simulink model "r2_deng_rev1_13_wide"  (R2012b)
settings: Solver=VariableStepDiscrete  StartTime=0.0  StopTime=2000  RelTol=1e-3
libraries: xbsIndex_r4 x7404, casper_library_sources x12, casper_library_misc x10, casper_library_communications x4, simulink x3, xps_library x2
(part 61 of 65)

== system r2_deng_rev1_13_wide/wng1/bus_mult/repb/bussify ==
  in1 : Inport
  in2 : Inport  Port=2
  in3 : Inport  Port=3
  in4 : Inport  Port=4
  in5 : Inport  Port=5
  in6 : Inport  Port=6
  in7 : Inport  Port=7
  in8 : Inport  Port=8
  concatenate : xbsIndex_r4/Concat  num_inputs=8  dbl_ovrd=off  block_type=concat
  reinterpret{1..8} (8 alike) : xbsIndex_r4/Reinterpret  force_arith_type=on  arith_type=Unsigned  force_bin_pt=on  bin_pt=0  block_type=reinterpret
      reinterpret1 settings: infoedit="Changes signal type without altering the binary representation.   You can changed the signal between signed and unsigned, and relocate the binary point.<br><br>Hardware notes: In hardware this block costs nothing.<br><br>Example:  Suppose the input is 6 bits wide, signed, with 2 fractional bits, and the output is forced to unsigned with 0 fractional bits.  Then an input of -2.0 (1110.00 in binary 2's complement) becomes an output of 56 (111000 in binary)."
  bus_out : Outport
  wires:
  concatenate/1 -> bus_out/1
  in1/1 -> reinterpret1/1
  reinterpret1/1 -> concatenate/1
  in2/1 -> reinterpret2/1
  reinterpret2/1 -> concatenate/2
  in3/1 -> reinterpret3/1
  reinterpret3/1 -> concatenate/3
  in4/1 -> reinterpret4/1
  reinterpret4/1 -> concatenate/4
  in5/1 -> reinterpret5/1
  reinterpret5/1 -> concatenate/5
  in6/1 -> reinterpret6/1
  reinterpret6/1 -> concatenate/6
  in7/1 -> reinterpret7/1
  reinterpret7/1 -> concatenate/7
  in8/1 -> reinterpret8/1
  reinterpret8/1 -> concatenate/8

== system r2_deng_rev1_13_wide/wng1/wgn1/tt800_uprng/tt800_engine ==
  note: Delay by (n - m - 3)
  note: Delay by (m)
  seed : Inport
  seed_en : Inport  Port=2
  Constant3 : xbsIndex_r4/Constant  const=0  gui_display_data_type=Fixed-point  arith_type=Unsigned  n_bits=32  bin_pt=0  preci_type=Single  exp_width=8  frac_width=24  explicit_period=off  period=1  equ=P=C  opselect=C  inp2=PCIN>>17  opr=+  inp1=P  carry=CIN  dbl_ovrd=off  block_type=constant
  Gateway Out{1..4} (4 alike) : xbsIndex_r4/Gateway Out  inherit_from_input=off  hdl_port=off  timing_constraint=None  locs_specified=off  LOCs={}  UseAsDAC=off  DACChannel='1'  block_type=gatewayout
      settings: infoedit="Gateway out block.  Converts Xilinx fixed point inputs into ouputs of type Simulink integer, double, or fixed point.<P><P>Hardware notes:  In hardware these blocks become top level output ports or are discarded, depending on how they are configured."  xl_area=[0 0 0 0 0 0 0]  block_version=10.1.3
  Logical : xbsIndex_r4/Logical  logical_function=XOR  inputs=3  en=off  latency=1  precision=Full  arith_type=Unsigned  n_bits=8  bin_pt=2  align_bp=off  dbl_ovrd=off  block_type=logical
      settings: xl_area=[32 32 0 32 0 0 0]
  Mux : xbsIndex_r4/Mux  inputs=2  en=off  latency=1  precision=Full  arith_type="Signed  (2's comp)"  n_bits=8  bin_pt=2  quantization=Truncate  overflow=Wrap  dbl_ovrd=off  block_type=mux
      settings: xl_area=[16 32 0 32 0 0 0]
  Mux1 : xbsIndex_r4/Mux  inputs=2  en=off  latency=1  precision=Full  arith_type="Signed  (2's comp)"  n_bits=8  bin_pt=2  quantization=Truncate  overflow=Wrap  dbl_ovrd=off  block_type=mux
      settings: xl_area=[16 32 0 32 0 0 0]
  Scope : Scope  NumInputPorts=4
      settings: YMin=-5~-5~-5~-5  YMax=5~5~5~5
  a : xbsIndex_r4/Constant  const=hex2dec('8EBFD028')  gui_display_data_type=Fixed-point  arith_type=Unsigned  n_bits=32  bin_pt=0  preci_type=Single  exp_width=8  frac_width=24  explicit_period=off  period=1  equ=P=C  opselect=C  inp2=PCIN>>17  opr=+  inp1=P  carry=CIN  dbl_ovrd=off  block_type=constant
  delay : xbsIndex_r4/Delay  rst=off  infoeditControl=Selection of Reset will increase slice count due to use of real FFs and instead of SRLs  en=off  latency=1  dbl_ovrd=off  reg_retiming=off  block_type=delay
      settings: xl_area=[16 32 0 0 0 0 0]
  lsb : xbsIndex_r4/Slice  nbits=1  boolean_output=off  mode=Lower Bit Location + Width  bit1=0  base1=MSB of Input  bit0=0  base0=LSB of Input  dbl_ovrd=off  block_type=slice
      settings: infoedit="Extracts a given range of bits from each input sample and presents it at the output.  The output type is ordinarily unsigned with binary point at zero, but can be Boolean when the slice is one bit wide.<P><P>Hardware notes: In hardware this block costs nothing."  block_version=10.1.3
  output : Subsystem
  rshift_1 : xbsIndex_r4/Shift  shift_dir=Right  shift_bits=1  en=off  latency=1  precision=User Defined  arith_type=Unsigned  n_bits=32  bin_pt=0  quantization=Truncate  overflow=Wrap  dbl_ovrd=off  block_type=shift
      settings: xl_area=[0 32 0 0 0 0 0]  block_version=10.1.3
  x_l : xbsIndex_r4/Delay  rst=off  infoeditControl=Selection of Reset will increase slice count due to use of real FFs and instead of SRLs  en=off  latency=7  dbl_ovrd=off  reg_retiming=off  block_type=delay
      settings: xl_area=[16 32 0 32 0 0 0]
  x_l_m : xbsIndex_r4/Delay  rst=off  infoeditControl=Selection of Reset will increase slice count due to use of real FFs and instead of SRLs  en=off  latency=25-7-3  dbl_ovrd=off  reg_retiming=off  block_type=delay
      settings: xl_area=[16 32 0 32 0 0 0]
  u : Outport
  wires:
  delay/1 -> Logical/1
  output/1(out) -> u/1
  Gateway Out3/1 -> Scope/4
  Gateway Out2/1 -> Scope/3
  Gateway Out4/1 -> Scope/2
  Gateway Out1/1 -> Scope/1
  seed/1 -> Mux1/3, Gateway Out4/1
  seed_en/1 -> Mux1/1, Gateway Out1/1
  Mux1/1 -> Gateway Out2/1, x_l_m/1
  Logical/1 -> Mux1/2, Gateway Out3/1
  Mux/1 -> Logical/3
  rshift_1/1 -> Logical/2
  a/1 -> Mux/3
  Constant3/1 -> Mux/2
  lsb/1 -> Mux/1
  x_l/1 -> output/1(in), rshift_1/1, lsb/1
  x_l_m/1 -> delay/1, x_l/1

== system r2_deng_rev1_13_wide/wng1/wgn1/tt800_uprng/tt800_seed_gen ==
  seed_in : Inport
  ld : Inport  Port=2
  rst : Inport  Port=3
  Expression : xbsIndex_r4/Expression  expression=(bootstrap | ld | ld_ext)  align_bp=on  en=off  latency=1  precision=Full  arith_type=Unsigned  n_bits=8  bin_pt=2  dbl_ovrd=off  block_type=expr
      settings: xl_area=[0, 0, 0, 0, 0, 0, 0]  block_version=10.1.3
  LFSR : xbsIndex_r4/LFSR  lfsr_type=Fibonacci  gate_type=XOR  n_bits=32  polynomial='C0000401'  rst_value='65498732'  rst=on  en=off  reloadable_seed=on  input_type=on  output_type=on  arith_type=Unsigned  bin_pt=0  dbl_ovrd=off  explicit_period=on  period=1  block_type=lfsr
      settings: xl_area=[17 32 0 33 0 0 0]  block_version=10.1.3
  bootstrap : Subsystem
  p24_extender : Subsystem
  pipeline1 : Subsystem  AncestorBlock=casper_library_delays/pipeline  mask(pipeline){latency=2}
      mask help:
      | An explicitly laid-out delay line to avoid mapping to SRL16s
      | for use in pipelining to help achieve timing closure.
      mask init:
      | pipeline_init(gcb,'latency',latency);
      settings: AttributesFormatString=Latency = %<latency>
      mask Display:
      | port_label('input', 1, 'd');
      | port_label('output', 1, 'q');
      | disp(['Z^-', num2str(latency)]);
  pipeline2 : Subsystem  AncestorBlock=casper_library_delays/pipeline  mask(pipeline){latency=2}
      mask help:
      | An explicitly laid-out delay line to avoid mapping to SRL16s
      | for use in pipelining to help achieve timing closure.
      mask init:
      | pipeline_init(gcb,'latency',latency);
      settings: AttributesFormatString=Latency = %<latency>
      mask Display:
      | port_label('input', 1, 'd');
      | port_label('output', 1, 'q');
      | disp(['Z^-', num2str(latency)]);
  r_edge_detect : Subsystem
  seed_out : Outport
  seed_en : Outport  Port=2
  wires:
  r_edge_detect/1(out) -> p24_extender/1(in)
  ld/1 -> LFSR/2, r_edge_detect/1(in), Expression/2
  Expression/1 -> seed_en/1
  seed_in/1 -> LFSR/1
  LFSR/1 -> seed_out/1
  bootstrap/1(out) -> Expression/1
  p24_extender/1(out) -> Expression/3
  rst/1 -> LFSR/3, pipeline2/1(d), pipeline1/1(d)
  pipeline2/1(q) -> p24_extender/2(rst)
  pipeline1/1(q) -> bootstrap/1(rst)

== system r2_deng_rev1_13_wide/wng1/wgn2/tt800_uprng/tt800_engine ==
  note: Delay by (n - m - 3)
  note: Delay by (m)
  seed : Inport
  seed_en : Inport  Port=2
  Constant3 : xbsIndex_r4/Constant  const=0  gui_display_data_type=Fixed-point  arith_type=Unsigned  n_bits=32  bin_pt=0  preci_type=Single  exp_width=8  frac_width=24  explicit_period=off  period=1  equ=P=C  opselect=C  inp2=PCIN>>17  opr=+  inp1=P  carry=CIN  dbl_ovrd=off  block_type=constant
  Gateway Out{1..4} (4 alike) : xbsIndex_r4/Gateway Out  inherit_from_input=off  hdl_port=off  timing_constraint=None  locs_specified=off  LOCs={}  UseAsDAC=off  DACChannel='1'  block_type=gatewayout
      settings: infoedit="Gateway out block.  Converts Xilinx fixed point inputs into ouputs of type Simulink integer, double, or fixed point.<P><P>Hardware notes:  In hardware these blocks become top level output ports or are discarded, depending on how they are configured."  xl_area=[0 0 0 0 0 0 0]  block_version=10.1.3
  Logical : xbsIndex_r4/Logical  logical_function=XOR  inputs=3  en=off  latency=1  precision=Full  arith_type=Unsigned  n_bits=8  bin_pt=2  align_bp=off  dbl_ovrd=off  block_type=logical
      settings: xl_area=[32 32 0 32 0 0 0]
  Mux : xbsIndex_r4/Mux  inputs=2  en=off  latency=1  precision=Full  arith_type="Signed  (2's comp)"  n_bits=8  bin_pt=2  quantization=Truncate  overflow=Wrap  dbl_ovrd=off  block_type=mux
      settings: xl_area=[16 32 0 32 0 0 0]
  Mux1 : xbsIndex_r4/Mux  inputs=2  en=off  latency=1  precision=Full  arith_type="Signed  (2's comp)"  n_bits=8  bin_pt=2  quantization=Truncate  overflow=Wrap  dbl_ovrd=off  block_type=mux
      settings: xl_area=[16 32 0 32 0 0 0]
  Scope : Scope  NumInputPorts=4
      settings: YMin=-5~-5~-5~-5  YMax=5~5~5~5
  a : xbsIndex_r4/Constant  const=hex2dec('8EBFD028')  gui_display_data_type=Fixed-point  arith_type=Unsigned  n_bits=32  bin_pt=0  preci_type=Single  exp_width=8  frac_width=24  explicit_period=off  period=1  equ=P=C  opselect=C  inp2=PCIN>>17  opr=+  inp1=P  carry=CIN  dbl_ovrd=off  block_type=constant
  delay : xbsIndex_r4/Delay  rst=off  infoeditControl=Selection of Reset will increase slice count due to use of real FFs and instead of SRLs  en=off  latency=1  dbl_ovrd=off  reg_retiming=off  block_type=delay
      settings: xl_area=[16 32 0 0 0 0 0]
  lsb : xbsIndex_r4/Slice  nbits=1  boolean_output=off  mode=Lower Bit Location + Width  bit1=0  base1=MSB of Input  bit0=0  base0=LSB of Input  dbl_ovrd=off  block_type=slice
      settings: infoedit="Extracts a given range of bits from each input sample and presents it at the output.  The output type is ordinarily unsigned with binary point at zero, but can be Boolean when the slice is one bit wide.<P><P>Hardware notes: In hardware this block costs nothing."  block_version=10.1.3
  output : Subsystem
  rshift_1 : xbsIndex_r4/Shift  shift_dir=Right  shift_bits=1  en=off  latency=1  precision=User Defined  arith_type=Unsigned  n_bits=32  bin_pt=0  quantization=Truncate  overflow=Wrap  dbl_ovrd=off  block_type=shift
      settings: xl_area=[0 32 0 0 0 0 0]  block_version=10.1.3
  x_l : xbsIndex_r4/Delay  rst=off  infoeditControl=Selection of Reset will increase slice count due to use of real FFs and instead of SRLs  en=off  latency=7  dbl_ovrd=off  reg_retiming=off  block_type=delay
      settings: xl_area=[16 32 0 32 0 0 0]
  x_l_m : xbsIndex_r4/Delay  rst=off  infoeditControl=Selection of Reset will increase slice count due to use of real FFs and instead of SRLs  en=off  latency=25-7-3  dbl_ovrd=off  reg_retiming=off  block_type=delay
      settings: xl_area=[16 32 0 32 0 0 0]
  u : Outport
  wires:
  delay/1 -> Logical/1
  output/1(out) -> u/1
  Gateway Out3/1 -> Scope/4
  Gateway Out2/1 -> Scope/3
  Gateway Out4/1 -> Scope/2
  Gateway Out1/1 -> Scope/1
  seed/1 -> Mux1/3, Gateway Out4/1
  seed_en/1 -> Mux1/1, Gateway Out1/1
  Mux1/1 -> Gateway Out2/1, x_l_m/1
  Logical/1 -> Mux1/2, Gateway Out3/1
  Mux/1 -> Logical/3
  rshift_1/1 -> Logical/2
  a/1 -> Mux/3
  Constant3/1 -> Mux/2
  lsb/1 -> Mux/1
  x_l/1 -> output/1(in), rshift_1/1, lsb/1
  x_l_m/1 -> delay/1, x_l/1

== system r2_deng_rev1_13_wide/wng1/wgn2/tt800_uprng/tt800_seed_gen ==
  seed_in : Inport
  ld : Inport  Port=2
  rst : Inport  Port=3
  Expression : xbsIndex_r4/Expression  expression=(bootstrap | ld | ld_ext)  align_bp=on  en=off  latency=1  precision=Full  arith_type=Unsigned  n_bits=8  bin_pt=2  dbl_ovrd=off  block_type=expr
      settings: xl_area=[0, 0, 0, 0, 0, 0, 0]  block_version=10.1.3
  LFSR : xbsIndex_r4/LFSR  lfsr_type=Fibonacci  gate_type=XOR  n_bits=32  polynomial='C0000401'  rst_value='32198754'  rst=on  en=off  reloadable_seed=on  input_type=on  output_type=on  arith_type=Unsigned  bin_pt=0  dbl_ovrd=off  explicit_period=on  period=1  block_type=lfsr
      settings: xl_area=[17 32 0 33 0 0 0]  block_version=10.1.3
  bootstrap : Subsystem
  p24_extender : Subsystem
  pipeline1 : Subsystem  AncestorBlock=casper_library_delays/pipeline  mask(pipeline){latency=2}
      mask help:
      | An explicitly laid-out delay line to avoid mapping to SRL16s
      | for use in pipelining to help achieve timing closure.
      mask init:
      | pipeline_init(gcb,'latency',latency);
      settings: AttributesFormatString=Latency = %<latency>
      mask Display:
      | port_label('input', 1, 'd');
      | port_label('output', 1, 'q');
      | disp(['Z^-', num2str(latency)]);
  pipeline2 : Subsystem  AncestorBlock=casper_library_delays/pipeline  mask(pipeline){latency=2}
      mask help:
      | An explicitly laid-out delay line to avoid mapping to SRL16s
      | for use in pipelining to help achieve timing closure.
      mask init:
      | pipeline_init(gcb,'latency',latency);
      settings: AttributesFormatString=Latency = %<latency>
      mask Display:
      | port_label('input', 1, 'd');
      | port_label('output', 1, 'q');
      | disp(['Z^-', num2str(latency)]);
  r_edge_detect : Subsystem
  seed_out : Outport
  seed_en : Outport  Port=2
  wires:
  r_edge_detect/1(out) -> p24_extender/1(in)
  ld/1 -> LFSR/2, r_edge_detect/1(in), Expression/2
  Expression/1 -> seed_en/1
  seed_in/1 -> LFSR/1
  LFSR/1 -> seed_out/1
  bootstrap/1(out) -> Expression/1
  p24_extender/1(out) -> Expression/3
  rst/1 -> pipeline1/1(d), pipeline2/1(d), LFSR/3
  pipeline1/1(q) -> p24_extender/2(rst)
  pipeline2/1(q) -> bootstrap/1(rst)

== system r2_deng_rev1_13_wide/wng1/wgn3/tt800_uprng/tt800_engine ==
  note: Delay by (n - m - 3)
  note: Delay by (m)
  seed : Inport
  seed_en : Inport  Port=2
  Constant3 : xbsIndex_r4/Constant  const=0  gui_display_data_type=Fixed-point  arith_type=Unsigned  n_bits=32  bin_pt=0  preci_type=Single  exp_width=8  frac_width=24  explicit_period=off  period=1  equ=P=C  opselect=C  inp2=PCIN>>17  opr=+  inp1=P  carry=CIN  dbl_ovrd=off  block_type=constant
  Gateway Out{1..4} (4 alike) : xbsIndex_r4/Gateway Out  inherit_from_input=off  hdl_port=off  timing_constraint=None  locs_specified=off  LOCs={}  UseAsDAC=off  DACChannel='1'  block_type=gatewayout
      settings: infoedit="Gateway out block.  Converts Xilinx fixed point inputs into ouputs of type Simulink integer, double, or fixed point.<P><P>Hardware notes:  In hardware these blocks become top level output ports or are discarded, depending on how they are configured."  xl_area=[0 0 0 0 0 0 0]  block_version=10.1.3
  Logical : xbsIndex_r4/Logical  logical_function=XOR  inputs=3  en=off  latency=1  precision=Full  arith_type=Unsigned  n_bits=8  bin_pt=2  align_bp=off  dbl_ovrd=off  block_type=logical
      settings: xl_area=[32 32 0 32 0 0 0]
  Mux : xbsIndex_r4/Mux  inputs=2  en=off  latency=1  precision=Full  arith_type="Signed  (2's comp)"  n_bits=8  bin_pt=2  quantization=Truncate  overflow=Wrap  dbl_ovrd=off  block_type=mux
      settings: xl_area=[16 32 0 32 0 0 0]
  Mux1 : xbsIndex_r4/Mux  inputs=2  en=off  latency=1  precision=Full  arith_type="Signed  (2's comp)"  n_bits=8  bin_pt=2  quantization=Truncate  overflow=Wrap  dbl_ovrd=off  block_type=mux
      settings: xl_area=[16 32 0 32 0 0 0]
  Scope : Scope  NumInputPorts=4
      settings: YMin=-5~-5~-5~-5  YMax=5~5~5~5
  a : xbsIndex_r4/Constant  const=hex2dec('8EBFD028')  gui_display_data_type=Fixed-point  arith_type=Unsigned  n_bits=32  bin_pt=0  preci_type=Single  exp_width=8  frac_width=24  explicit_period=off  period=1  equ=P=C  opselect=C  inp2=PCIN>>17  opr=+  inp1=P  carry=CIN  dbl_ovrd=off  block_type=constant
  delay : xbsIndex_r4/Delay  rst=off  infoeditControl=Selection of Reset will increase slice count due to use of real FFs and instead of SRLs  en=off  latency=1  dbl_ovrd=off  reg_retiming=off  block_type=delay
      settings: xl_area=[16 32 0 0 0 0 0]
  lsb : xbsIndex_r4/Slice  nbits=1  boolean_output=off  mode=Lower Bit Location + Width  bit1=0  base1=MSB of Input  bit0=0  base0=LSB of Input  dbl_ovrd=off  block_type=slice
      settings: infoedit="Extracts a given range of bits from each input sample and presents it at the output.  The output type is ordinarily unsigned with binary point at zero, but can be Boolean when the slice is one bit wide.<P><P>Hardware notes: In hardware this block costs nothing."  block_version=10.1.3
  output : Subsystem
  rshift_1 : xbsIndex_r4/Shift  shift_dir=Right  shift_bits=1  en=off  latency=1  precision=User Defined  arith_type=Unsigned  n_bits=32  bin_pt=0  quantization=Truncate  overflow=Wrap  dbl_ovrd=off  block_type=shift
      settings: xl_area=[0 32 0 0 0 0 0]  block_version=10.1.3
  x_l : xbsIndex_r4/Delay  rst=off  infoeditControl=Selection of Reset will increase slice count due to use of real FFs and instead of SRLs  en=off  latency=7  dbl_ovrd=off  reg_retiming=off  block_type=delay
      settings: xl_area=[16 32 0 32 0 0 0]
  x_l_m : xbsIndex_r4/Delay  rst=off  infoeditControl=Selection of Reset will increase slice count due to use of real FFs and instead of SRLs  en=off  latency=25-7-3  dbl_ovrd=off  reg_retiming=off  block_type=delay
      settings: xl_area=[16 32 0 32 0 0 0]
  u : Outport
  wires:
  delay/1 -> Logical/1
  output/1(out) -> u/1
  Gateway Out3/1 -> Scope/4
  Gateway Out2/1 -> Scope/3
  Gateway Out4/1 -> Scope/2
  Gateway Out1/1 -> Scope/1
  seed/1 -> Mux1/3, Gateway Out4/1
  seed_en/1 -> Mux1/1, Gateway Out1/1
  Mux1/1 -> Gateway Out2/1, x_l_m/1
  Logical/1 -> Mux1/2, Gateway Out3/1
  Mux/1 -> Logical/3
  rshift_1/1 -> Logical/2
  a/1 -> Mux/3
  Constant3/1 -> Mux/2
  lsb/1 -> Mux/1
  x_l/1 -> output/1(in), rshift_1/1, lsb/1
  x_l_m/1 -> delay/1, x_l/1

== system r2_deng_rev1_13_wide/wng1/wgn3/tt800_uprng/tt800_seed_gen ==
  seed_in : Inport
  ld : Inport  Port=2
  rst : Inport  Port=3
  Expression : xbsIndex_r4/Expression  expression=(bootstrap | ld | ld_ext)  align_bp=on  en=off  latency=1  precision=Full  arith_type=Unsigned  n_bits=8  bin_pt=2  dbl_ovrd=off  block_type=expr
      settings: xl_area=[0, 0, 0, 0, 0, 0, 0]  block_version=10.1.3
  LFSR : xbsIndex_r4/LFSR  lfsr_type=Fibonacci  gate_type=XOR  n_bits=32  polynomial='C0000401'  rst_value='45612378'  rst=on  en=off  reloadable_seed=on  input_type=on  output_type=on  arith_type=Unsigned  bin_pt=0  dbl_ovrd=off  explicit_period=on  period=1  block_type=lfsr
      settings: xl_area=[17 32 0 33 0 0 0]  block_version=10.1.3
  bootstrap : Subsystem
  p24_extender : Subsystem
  pipeline1 : Subsystem  AncestorBlock=casper_library_delays/pipeline  mask(pipeline){latency=2}
      mask help:
      | An explicitly laid-out delay line to avoid mapping to SRL16s
      | for use in pipelining to help achieve timing closure.
      mask init:
      | pipeline_init(gcb,'latency',latency);
      settings: AttributesFormatString=Latency = %<latency>
      mask Display:
      | port_label('input', 1, 'd');
      | port_label('output', 1, 'q');
      | disp(['Z^-', num2str(latency)]);
  pipeline2 : Subsystem  AncestorBlock=casper_library_delays/pipeline  mask(pipeline){latency=2}
      mask help:
      | An explicitly laid-out delay line to avoid mapping to SRL16s
      | for use in pipelining to help achieve timing closure.
      mask init:
      | pipeline_init(gcb,'latency',latency);
      settings: AttributesFormatString=Latency = %<latency>
      mask Display:
      | port_label('input', 1, 'd');
      | port_label('output', 1, 'q');
      | disp(['Z^-', num2str(latency)]);
  r_edge_detect : Subsystem
  seed_out : Outport
  seed_en : Outport  Port=2
  wires:
  r_edge_detect/1(out) -> p24_extender/1(in)
  ld/1 -> LFSR/2, r_edge_detect/1(in), Expression/2
  Expression/1 -> seed_en/1
  seed_in/1 -> LFSR/1
  LFSR/1 -> seed_out/1
  bootstrap/1(out) -> Expression/1
  p24_extender/1(out) -> Expression/3
  rst/1 -> pipeline1/1(d), pipeline2/1(d), LFSR/3
  pipeline1/1(q) -> p24_extender/2(rst)
  pipeline2/1(q) -> bootstrap/1(rst)

== system r2_deng_rev1_13_wide/wng1/wgn4/tt800_uprng/tt800_engine ==
  note: Delay by (n - m - 3)
  note: Delay by (m)
  seed : Inport
  seed_en : Inport  Port=2
  Constant3 : xbsIndex_r4/Constant  const=0  gui_display_data_type=Fixed-point  arith_type=Unsigned  n_bits=32  bin_pt=0  preci_type=Single  exp_width=8  frac_width=24  explicit_period=off  period=1  equ=P=C  opselect=C  inp2=PCIN>>17  opr=+  inp1=P  carry=CIN  dbl_ovrd=off  block_type=constant
  Gateway Out{1..4} (4 alike) : xbsIndex_r4/Gateway Out  inherit_from_input=off  hdl_port=off  timing_constraint=None  locs_specified=off  LOCs={}  UseAsDAC=off  DACChannel='1'  block_type=gatewayout
      settings: infoedit="Gateway out block.  Converts Xilinx fixed point inputs into ouputs of type Simulink integer, double, or fixed point.<P><P>Hardware notes:  In hardware these blocks become top level output ports or are discarded, depending on how they are configured."  xl_area=[0 0 0 0 0 0 0]  block_version=10.1.3
  Logical : xbsIndex_r4/Logical  logical_function=XOR  inputs=3  en=off  latency=1  precision=Full  arith_type=Unsigned  n_bits=8  bin_pt=2  align_bp=off  dbl_ovrd=off  block_type=logical
      settings: xl_area=[32 32 0 32 0 0 0]
  Mux : xbsIndex_r4/Mux  inputs=2  en=off  latency=1  precision=Full  arith_type="Signed  (2's comp)"  n_bits=8  bin_pt=2  quantization=Truncate  overflow=Wrap  dbl_ovrd=off  block_type=mux
      settings: xl_area=[16 32 0 32 0 0 0]
  Mux1 : xbsIndex_r4/Mux  inputs=2  en=off  latency=1  precision=Full  arith_type="Signed  (2's comp)"  n_bits=8  bin_pt=2  quantization=Truncate  overflow=Wrap  dbl_ovrd=off  block_type=mux
      settings: xl_area=[16 32 0 32 0 0 0]
  Scope : Scope  NumInputPorts=4
      settings: YMin=-5~-5~-5~-5  YMax=5~5~5~5
  a : xbsIndex_r4/Constant  const=hex2dec('8EBFD028')  gui_display_data_type=Fixed-point  arith_type=Unsigned  n_bits=32  bin_pt=0  preci_type=Single  exp_width=8  frac_width=24  explicit_period=off  period=1  equ=P=C  opselect=C  inp2=PCIN>>17  opr=+  inp1=P  carry=CIN  dbl_ovrd=off  block_type=constant
  delay : xbsIndex_r4/Delay  rst=off  infoeditControl=Selection of Reset will increase slice count due to use of real FFs and instead of SRLs  en=off  latency=1  dbl_ovrd=off  reg_retiming=off  block_type=delay
      settings: xl_area=[16 32 0 0 0 0 0]
  lsb : xbsIndex_r4/Slice  nbits=1  boolean_output=off  mode=Lower Bit Location + Width  bit1=0  base1=MSB of Input  bit0=0  base0=LSB of Input  dbl_ovrd=off  block_type=slice
      settings: infoedit="Extracts a given range of bits from each input sample and presents it at the output.  The output type is ordinarily unsigned with binary point at zero, but can be Boolean when the slice is one bit wide.<P><P>Hardware notes: In hardware this block costs nothing."  block_version=10.1.3
  output : Subsystem
  rshift_1 : xbsIndex_r4/Shift  shift_dir=Right  shift_bits=1  en=off  latency=1  precision=User Defined  arith_type=Unsigned  n_bits=32  bin_pt=0  quantization=Truncate  overflow=Wrap  dbl_ovrd=off  block_type=shift
      settings: xl_area=[0 32 0 0 0 0 0]  block_version=10.1.3
  x_l : xbsIndex_r4/Delay  rst=off  infoeditControl=Selection of Reset will increase slice count due to use of real FFs and instead of SRLs  en=off  latency=7  dbl_ovrd=off  reg_retiming=off  block_type=delay
      settings: xl_area=[16 32 0 32 0 0 0]
  x_l_m : xbsIndex_r4/Delay  rst=off  infoeditControl=Selection of Reset will increase slice count due to use of real FFs and instead of SRLs  en=off  latency=25-7-3  dbl_ovrd=off  reg_retiming=off  block_type=delay
      settings: xl_area=[16 32 0 32 0 0 0]
  u : Outport
  wires:
  delay/1 -> Logical/1
  output/1(out) -> u/1
  Gateway Out3/1 -> Scope/4
  Gateway Out2/1 -> Scope/3
  Gateway Out4/1 -> Scope/2
  Gateway Out1/1 -> Scope/1
  seed/1 -> Mux1/3, Gateway Out4/1
  seed_en/1 -> Mux1/1, Gateway Out1/1
  Mux1/1 -> Gateway Out2/1, x_l_m/1
  Logical/1 -> Mux1/2, Gateway Out3/1
  Mux/1 -> Logical/3
  rshift_1/1 -> Logical/2
  a/1 -> Mux/3
  Constant3/1 -> Mux/2
  lsb/1 -> Mux/1
  x_l/1 -> output/1(in), rshift_1/1, lsb/1
  x_l_m/1 -> delay/1, x_l/1

== system r2_deng_rev1_13_wide/wng1/wgn4/tt800_uprng/tt800_seed_gen ==
  seed_in : Inport
  ld : Inport  Port=2
  rst : Inport  Port=3
  Expression : xbsIndex_r4/Expression  expression=(bootstrap | ld | ld_ext)  align_bp=on  en=off  latency=1  precision=Full  arith_type=Unsigned  n_bits=8  bin_pt=2  dbl_ovrd=off  block_type=expr
      settings: xl_area=[0, 0, 0, 0, 0, 0, 0]  block_version=10.1.3
  LFSR : xbsIndex_r4/LFSR  lfsr_type=Fibonacci  gate_type=XOR  n_bits=32  polynomial='C0000401'  rst_value='74563218'  rst=on  en=off  reloadable_seed=on  input_type=on  output_type=on  arith_type=Unsigned  bin_pt=0  dbl_ovrd=off  explicit_period=on  period=1  block_type=lfsr
      settings: xl_area=[17 32 0 33 0 0 0]  block_version=10.1.3
  bootstrap : Subsystem
  p24_extender : Subsystem
  pipeline1 : Subsystem  AncestorBlock=casper_library_delays/pipeline  mask(pipeline){latency=2}
      mask help:
      | An explicitly laid-out delay line to avoid mapping to SRL16s
      | for use in pipelining to help achieve timing closure.
      mask init:
      | pipeline_init(gcb,'latency',latency);
      settings: AttributesFormatString=Latency = %<latency>
      mask Display:
      | port_label('input', 1, 'd');
      | port_label('output', 1, 'q');
      | disp(['Z^-', num2str(latency)]);
  pipeline2 : Subsystem  AncestorBlock=casper_library_delays/pipeline  mask(pipeline){latency=2}
      mask help:
      | An explicitly laid-out delay line to avoid mapping to SRL16s
      | for use in pipelining to help achieve timing closure.
      mask init:
      | pipeline_init(gcb,'latency',latency);
      settings: AttributesFormatString=Latency = %<latency>
      mask Display:
      | port_label('input', 1, 'd');
      | port_label('output', 1, 'q');
      | disp(['Z^-', num2str(latency)]);
  r_edge_detect : Subsystem
  seed_out : Outport
  seed_en : Outport  Port=2
  wires:
  r_edge_detect/1(out) -> p24_extender/1(in)
  ld/1 -> LFSR/2, r_edge_detect/1(in), Expression/2
  Expression/1 -> seed_en/1
  seed_in/1 -> LFSR/1
  LFSR/1 -> seed_out/1
  bootstrap/1(out) -> Expression/1
  p24_extender/1(out) -> Expression/3
  rst/1 -> LFSR/3, pipeline1/1(d), pipeline2/1(d)
  pipeline1/1(q) -> p24_extender/2(rst)
  pipeline2/1(q) -> bootstrap/1(rst)

== system r2_deng_rev1_13_wide/wng_corr/bus_mult/repa/bussify ==
  in1 : Inport
  reinterpret1 : xbsIndex_r4/Reinterpret  force_arith_type=on  arith_type=Unsigned  force_bin_pt=on  bin_pt=0  block_type=reinterpret
      settings: infoedit="Changes signal type without altering the binary representation.   You can changed the signal between signed and unsigned, and relocate the binary point.<br><br>Hardware notes: In hardware this block costs nothing.<br><br>Example:  Suppose the input is 6 bits wide, signed, with 2 fractional bits, and the output is forced to unsigned with 0 fractional bits.  Then an input of -2.0 (1110.00 in binary 2's complement) becomes an output of 56 (111000 in binary)."
  bus_out : Outport
  wires:
  in1/1 -> reinterpret1/1
  reinterpret1/1 -> bus_out/1

== system r2_deng_rev1_13_wide/wng_corr/bus_mult/repb/bussify ==
  in1 : Inport
  in2 : Inport  Port=2
  in3 : Inport  Port=3
  in4 : Inport  Port=4
  in5 : Inport  Port=5
  in6 : Inport  Port=6
  in7 : Inport  Port=7
  in8 : Inport  Port=8
  concatenate : xbsIndex_r4/Concat  num_inputs=8  dbl_ovrd=off  block_type=concat
  reinterpret{1..8} (8 alike) : xbsIndex_r4/Reinterpret  force_arith_type=on  arith_type=Unsigned  force_bin_pt=on  bin_pt=0  block_type=reinterpret
      reinterpret1 settings: infoedit="Changes signal type without altering the binary representation.   You can changed the signal between signed and unsigned, and relocate the binary point.<br><br>Hardware notes: In hardware this block costs nothing.<br><br>Example:  Suppose the input is 6 bits wide, signed, with 2 fractional bits, and the output is forced to unsigned with 0 fractional bits.  Then an input of -2.0 (1110.00 in binary 2's complement) becomes an output of 56 (111000 in binary)."
  bus_out : Outport
  wires:
  concatenate/1 -> bus_out/1
  in1/1 -> reinterpret1/1
  reinterpret1/1 -> concatenate/1
  in2/1 -> reinterpret2/1
  reinterpret2/1 -> concatenate/2
  in3/1 -> reinterpret3/1
  reinterpret3/1 -> concatenate/3
  in4/1 -> reinterpret4/1
  reinterpret4/1 -> concatenate/4
  in5/1 -> reinterpret5/1
  reinterpret5/1 -> concatenate/5
  in6/1 -> reinterpret6/1
  reinterpret6/1 -> concatenate/6
  in7/1 -> reinterpret7/1
  reinterpret7/1 -> concatenate/7
  in8/1 -> reinterpret8/1
  reinterpret8/1 -> concatenate/8

== system r2_deng_rev1_13_wide/wng_corr/wgn1/tt800_uprng/tt800_engine ==
  note: Delay by (n - m - 3)
  note: Delay by (m)
  seed : Inport
  seed_en : Inport  Port=2
  Constant3 : xbsIndex_r4/Constant  const=0  gui_display_data_type=Fixed-point  arith_type=Unsigned  n_bits=32  bin_pt=0  preci_type=Single  exp_width=8  frac_width=24  explicit_period=off  period=1  equ=P=C  opselect=C  inp2=PCIN>>17  opr=+  inp1=P  carry=CIN  dbl_ovrd=off  block_type=constant
  Gateway Out{1..4} (4 alike) : xbsIndex_r4/Gateway Out  inherit_from_input=off  hdl_port=off  timing_constraint=None  locs_specified=off  LOCs={}  UseAsDAC=off  DACChannel='1'  block_type=gatewayout
      settings: infoedit="Gateway out block.  Converts Xilinx fixed point inputs into ouputs of type Simulink integer, double, or fixed point.<P><P>Hardware notes:  In hardware these blocks become top level output ports or are discarded, depending on how they are configured."  xl_area=[0 0 0 0 0 0 0]  block_version=10.1.3
  Logical : xbsIndex_r4/Logical  logical_function=XOR  inputs=3  en=off  latency=1  precision=Full  arith_type=Unsigned  n_bits=8  bin_pt=2  align_bp=off  dbl_ovrd=off  block_type=logical
      settings: xl_area=[32 32 0 32 0 0 0]
  Mux : xbsIndex_r4/Mux  inputs=2  en=off  latency=1  precision=Full  arith_type="Signed  (2's comp)"  n_bits=8  bin_pt=2  quantization=Truncate  overflow=Wrap  dbl_ovrd=off  block_type=mux
      settings: xl_area=[16 32 0 32 0 0 0]
  Mux1 : xbsIndex_r4/Mux  inputs=2  en=off  latency=1  precision=Full  arith_type="Signed  (2's comp)"  n_bits=8  bin_pt=2  quantization=Truncate  overflow=Wrap  dbl_ovrd=off  block_type=mux
      settings: xl_area=[16 32 0 32 0 0 0]
  Scope : Scope  NumInputPorts=4
      settings: YMin=-5~-5~-5~-5  YMax=5~5~5~5
  a : xbsIndex_r4/Constant  const=hex2dec('8EBFD028')  gui_display_data_type=Fixed-point  arith_type=Unsigned  n_bits=32  bin_pt=0  preci_type=Single  exp_width=8  frac_width=24  explicit_period=off  period=1  equ=P=C  opselect=C  inp2=PCIN>>17  opr=+  inp1=P  carry=CIN  dbl_ovrd=off  block_type=constant
  delay : xbsIndex_r4/Delay  rst=off  infoeditControl=Selection of Reset will increase slice count due to use of real FFs and instead of SRLs  en=off  latency=1  dbl_ovrd=off  reg_retiming=off  block_type=delay
      settings: xl_area=[16 32 0 0 0 0 0]
  lsb : xbsIndex_r4/Slice  nbits=1  boolean_output=off  mode=Lower Bit Location + Width  bit1=0  base1=MSB of Input  bit0=0  base0=LSB of Input  dbl_ovrd=off  block_type=slice
      settings: infoedit="Extracts a given range of bits from each input sample and presents it at the output.  The output type is ordinarily unsigned with binary point at zero, but can be Boolean when the slice is one bit wide.<P><P>Hardware notes: In hardware this block costs nothing."  block_version=10.1.3
  output : Subsystem
  rshift_1 : xbsIndex_r4/Shift  shift_dir=Right  shift_bits=1  en=off  latency=1  precision=User Defined  arith_type=Unsigned  n_bits=32  bin_pt=0  quantization=Truncate  overflow=Wrap  dbl_ovrd=off  block_type=shift
      settings: xl_area=[0 32 0 0 0 0 0]  block_version=10.1.3
  x_l : xbsIndex_r4/Delay  rst=off  infoeditControl=Selection of Reset will increase slice count due to use of real FFs and instead of SRLs  en=off  latency=7  dbl_ovrd=off  reg_retiming=off  block_type=delay
      settings: xl_area=[16 32 0 32 0 0 0]
  x_l_m : xbsIndex_r4/Delay  rst=off  infoeditControl=Selection of Reset will increase slice count due to use of real FFs and instead of SRLs  en=off  latency=25-7-3  dbl_ovrd=off  reg_retiming=off  block_type=delay
      settings: xl_area=[16 32 0 32 0 0 0]
  u : Outport
  wires:
  delay/1 -> Logical/1
  output/1(out) -> u/1
  Gateway Out3/1 -> Scope/4
  Gateway Out2/1 -> Scope/3
  Gateway Out4/1 -> Scope/2
  Gateway Out1/1 -> Scope/1
  seed/1 -> Mux1/3, Gateway Out4/1
  seed_en/1 -> Mux1/1, Gateway Out1/1
  Mux1/1 -> Gateway Out2/1, x_l_m/1
  Logical/1 -> Mux1/2, Gateway Out3/1
  Mux/1 -> Logical/3
  rshift_1/1 -> Logical/2
  a/1 -> Mux/3
  Constant3/1 -> Mux/2
  lsb/1 -> Mux/1
  x_l/1 -> output/1(in), rshift_1/1, lsb/1
  x_l_m/1 -> delay/1, x_l/1

== system r2_deng_rev1_13_wide/wng_corr/wgn1/tt800_uprng/tt800_seed_gen ==
  seed_in : Inport
  ld : Inport  Port=2
  rst : Inport  Port=3
  Expression : xbsIndex_r4/Expression  expression=(bootstrap | ld | ld_ext)  align_bp=on  en=off  latency=1  precision=Full  arith_type=Unsigned  n_bits=8  bin_pt=2  dbl_ovrd=off  block_type=expr
      settings: xl_area=[0, 0, 0, 0, 0, 0, 0]  block_version=10.1.3
  Gateway Out : xbsIndex_r4/Gateway Out  inherit_from_input=off  hdl_port=on  timing_constraint=None  locs_specified=off  LOCs={}  UseAsDAC=off  DACChannel='1'  block_type=gatewayout
  Gateway Out1 : xbsIndex_r4/Gateway Out  inherit_from_input=off  hdl_port=on  timing_constraint=None  locs_specified=off  LOCs={}  UseAsDAC=off  DACChannel='1'  block_type=gatewayout
  LFSR : xbsIndex_r4/LFSR  lfsr_type=Fibonacci  gate_type=XOR  n_bits=32  polynomial='C0000401'  rst_value='75386429'  rst=on  en=off  reloadable_seed=on  input_type=on  output_type=on  arith_type=Unsigned  bin_pt=0  dbl_ovrd=off  explicit_period=on  period=1  block_type=lfsr
      settings: xl_area=[17 32 0 33 0 0 0]  block_version=10.1.3
  To Workspace : ToWorkspace  VariableName=seed_out  SampleTime=-1  SaveFormat=Timeseries
  To Workspace1 : ToWorkspace  VariableName=seed_en  SampleTime=-1  SaveFormat=Timeseries
  bootstrap : Subsystem
  p24_extender : Subsystem
  pipeline1 : Subsystem  AncestorBlock=casper_library_delays/pipeline  mask(pipeline){latency=2}
      mask help:
      | An explicitly laid-out delay line to avoid mapping to SRL16s
      | for use in pipelining to help achieve timing closure.
      mask init:
      | pipeline_init(gcb,'latency',latency);
      settings: AttributesFormatString=Latency = %<latency>
      mask Display:
      | port_label('input', 1, 'd');
      | port_label('output', 1, 'q');
      | disp(['Z^-', num2str(latency)]);
  pipeline2 : Subsystem  AncestorBlock=casper_library_delays/pipeline  mask(pipeline){latency=2}
      mask help:
      | An explicitly laid-out delay line to avoid mapping to SRL16s
      | for use in pipelining to help achieve timing closure.
      mask init:
      | pipeline_init(gcb,'latency',latency);
      settings: AttributesFormatString=Latency = %<latency>
      mask Display:
      | port_label('input', 1, 'd');
      | port_label('output', 1, 'q');
      | disp(['Z^-', num2str(latency)]);
  r_edge_detect : Subsystem
  seed_out : Outport
  seed_en : Outport  Port=2
  wires:
  r_edge_detect/1(out) -> p24_extender/1(in)
  ld/1 -> LFSR/2, r_edge_detect/1(in), Expression/2
  Expression/1 -> Gateway Out1/1, seed_en/1
  seed_in/1 -> LFSR/1
  LFSR/1 -> seed_out/1, Gateway Out/1
  bootstrap/1(out) -> Expression/1
  p24_extender/1(out) -> Expression/3
  rst/1 -> LFSR/3, pipeline2/1(d), pipeline1/1(d)
  Gateway Out/1 -> To Workspace/1
  Gateway Out1/1 -> To Workspace1/1
  pipeline2/1(q) -> p24_extender/2(rst)
  pipeline1/1(q) -> bootstrap/1(rst)

== system r2_deng_rev1_13_wide/wng_corr/wgn2/tt800_uprng/tt800_engine ==
  note: Delay by (n - m - 3)
  note: Delay by (m)
  seed : Inport
  seed_en : Inport  Port=2
  Constant3 : xbsIndex_r4/Constant  const=0  gui_display_data_type=Fixed-point  arith_type=Unsigned  n_bits=32  bin_pt=0  preci_type=Single  exp_width=8  frac_width=24  explicit_period=off  period=1  equ=P=C  opselect=C  inp2=PCIN>>17  opr=+  inp1=P  carry=CIN  dbl_ovrd=off  block_type=constant
  Gateway Out{1..4} (4 alike) : xbsIndex_r4/Gateway Out  inherit_from_input=off  hdl_port=off  timing_constraint=None  locs_specified=off  LOCs={}  UseAsDAC=off  DACChannel='1'  block_type=gatewayout
      settings: infoedit="Gateway out block.  Converts Xilinx fixed point inputs into ouputs of type Simulink integer, double, or fixed point.<P><P>Hardware notes:  In hardware these blocks become top level output ports or are discarded, depending on how they are configured."  xl_area=[0 0 0 0 0 0 0]  block_version=10.1.3
  Logical : xbsIndex_r4/Logical  logical_function=XOR  inputs=3  en=off  latency=1  precision=Full  arith_type=Unsigned  n_bits=8  bin_pt=2  align_bp=off  dbl_ovrd=off  block_type=logical
      settings: xl_area=[32 32 0 32 0 0 0]
  Mux : xbsIndex_r4/Mux  inputs=2  en=off  latency=1  precision=Full  arith_type="Signed  (2's comp)"  n_bits=8  bin_pt=2  quantization=Truncate  overflow=Wrap  dbl_ovrd=off  block_type=mux
      settings: xl_area=[16 32 0 32 0 0 0]
  Mux1 : xbsIndex_r4/Mux  inputs=2  en=off  latency=1  precision=Full  arith_type="Signed  (2's comp)"  n_bits=8  bin_pt=2  quantization=Truncate  overflow=Wrap  dbl_ovrd=off  block_type=mux
      settings: xl_area=[16 32 0 32 0 0 0]
  Scope : Scope  NumInputPorts=4
      settings: YMin=-5~-5~-5~-5  YMax=5~5~5~5
  a : xbsIndex_r4/Constant  const=hex2dec('8EBFD028')  gui_display_data_type=Fixed-point  arith_type=Unsigned  n_bits=32  bin_pt=0  preci_type=Single  exp_width=8  frac_width=24  explicit_period=off  period=1  equ=P=C  opselect=C  inp2=PCIN>>17  opr=+  inp1=P  carry=CIN  dbl_ovrd=off  block_type=constant
  delay : xbsIndex_r4/Delay  rst=off  infoeditControl=Selection of Reset will increase slice count due to use of real FFs and instead of SRLs  en=off  latency=1  dbl_ovrd=off  reg_retiming=off  block_type=delay
      settings: xl_area=[16 32 0 0 0 0 0]
  lsb : xbsIndex_r4/Slice  nbits=1  boolean_output=off  mode=Lower Bit Location + Width  bit1=0  base1=MSB of Input  bit0=0  base0=LSB of Input  dbl_ovrd=off  block_type=slice
      settings: infoedit="Extracts a given range of bits from each input sample and presents it at the output.  The output type is ordinarily unsigned with binary point at zero, but can be Boolean when the slice is one bit wide.<P><P>Hardware notes: In hardware this block costs nothing."  block_version=10.1.3
  output : Subsystem
  rshift_1 : xbsIndex_r4/Shift  shift_dir=Right  shift_bits=1  en=off  latency=1  precision=User Defined  arith_type=Unsigned  n_bits=32  bin_pt=0  quantization=Truncate  overflow=Wrap  dbl_ovrd=off  block_type=shift
      settings: xl_area=[0 32 0 0 0 0 0]  block_version=10.1.3
  x_l : xbsIndex_r4/Delay  rst=off  infoeditControl=Selection of Reset will increase slice count due to use of real FFs and instead of SRLs  en=off  latency=7  dbl_ovrd=off  reg_retiming=off  block_type=delay
      settings: xl_area=[16 32 0 32 0 0 0]
  x_l_m : xbsIndex_r4/Delay  rst=off  infoeditControl=Selection of Reset will increase slice count due to use of real FFs and instead of SRLs  en=off  latency=25-7-3  dbl_ovrd=off  reg_retiming=off  block_type=delay
      settings: xl_area=[16 32 0 32 0 0 0]
  u : Outport
  wires:
  delay/1 -> Logical/1
  output/1(out) -> u/1
  Gateway Out3/1 -> Scope/4
  Gateway Out2/1 -> Scope/3
  Gateway Out4/1 -> Scope/2
  Gateway Out1/1 -> Scope/1
  seed/1 -> Mux1/3, Gateway Out4/1
  seed_en/1 -> Mux1/1, Gateway Out1/1
  Mux1/1 -> Gateway Out2/1, x_l_m/1
  Logical/1 -> Mux1/2, Gateway Out3/1
  Mux/1 -> Logical/3
  rshift_1/1 -> Logical/2
  a/1 -> Mux/3
  Constant3/1 -> Mux/2
  lsb/1 -> Mux/1
  x_l/1 -> output/1(in), rshift_1/1, lsb/1
  x_l_m/1 -> delay/1, x_l/1

== system r2_deng_rev1_13_wide/wng_corr/wgn2/tt800_uprng/tt800_seed_gen ==
  seed_in : Inport
  ld : Inport  Port=2
  rst : Inport  Port=3
  Expression : xbsIndex_r4/Expression  expression=(bootstrap | ld | ld_ext)  align_bp=on  en=off  latency=1  precision=Full  arith_type=Unsigned  n_bits=8  bin_pt=2  dbl_ovrd=off  block_type=expr
      settings: xl_area=[0, 0, 0, 0, 0, 0, 0]  block_version=10.1.3
  LFSR : xbsIndex_r4/LFSR  lfsr_type=Fibonacci  gate_type=XOR  n_bits=32  polynomial='C0000401'  rst_value='95123754'  rst=on  en=off  reloadable_seed=on  input_type=on  output_type=on  arith_type=Unsigned  bin_pt=0  dbl_ovrd=off  explicit_period=on  period=1  block_type=lfsr
      settings: xl_area=[17 32 0 33 0 0 0]  block_version=10.1.3
  bootstrap : Subsystem
  p24_extender : Subsystem
  pipeline1 : Subsystem  AncestorBlock=casper_library_delays/pipeline  mask(pipeline){latency=2}
      mask help:
      | An explicitly laid-out delay line to avoid mapping to SRL16s
      | for use in pipelining to help achieve timing closure.
      mask init:
      | pipeline_init(gcb,'latency',latency);
      settings: AttributesFormatString=Latency = %<latency>
      mask Display:
      | port_label('input', 1, 'd');
      | port_label('output', 1, 'q');
      | disp(['Z^-', num2str(latency)]);
  pipeline2 : Subsystem  AncestorBlock=casper_library_delays/pipeline  mask(pipeline){latency=2}
      mask help:
      | An explicitly laid-out delay line to avoid mapping to SRL16s
      | for use in pipelining to help achieve timing closure.
      mask init:
      | pipeline_init(gcb,'latency',latency);
      settings: AttributesFormatString=Latency = %<latency>
      mask Display:
      | port_label('input', 1, 'd');
      | port_label('output', 1, 'q');
      | disp(['Z^-', num2str(latency)]);
  r_edge_detect : Subsystem
  seed_out : Outport
  seed_en : Outport  Port=2
  wires:
  r_edge_detect/1(out) -> p24_extender/1(in)
  ld/1 -> LFSR/2, r_edge_detect/1(in), Expression/2
  Expression/1 -> seed_en/1
  seed_in/1 -> LFSR/1
  LFSR/1 -> seed_out/1
  bootstrap/1(out) -> Expression/1
  p24_extender/1(out) -> Expression/3
  rst/1 -> pipeline1/1(d), pipeline2/1(d), LFSR/3
  pipeline1/1(q) -> p24_extender/2(rst)
  pipeline2/1(q) -> bootstrap/1(rst)

== system r2_deng_rev1_13_wide/wng_corr/wgn3/tt800_uprng/tt800_engine ==
  note: Delay by (n - m - 3)
  note: Delay by (m)
  seed : Inport
  seed_en : Inport  Port=2
  Constant3 : xbsIndex_r4/Constant  const=0  gui_display_data_type=Fixed-point  arith_type=Unsigned  n_bits=32  bin_pt=0  preci_type=Single  exp_width=8  frac_width=24  explicit_period=off  period=1  equ=P=C  opselect=C  inp2=PCIN>>17  opr=+  inp1=P  carry=CIN  dbl_ovrd=off  block_type=constant
  Gateway Out{1..4} (4 alike) : xbsIndex_r4/Gateway Out  inherit_from_input=off  hdl_port=off  timing_constraint=None  locs_specified=off  LOCs={}  UseAsDAC=off  DACChannel='1'  block_type=gatewayout
      settings: infoedit="Gateway out block.  Converts Xilinx fixed point inputs into ouputs of type Simulink integer, double, or fixed point.<P><P>Hardware notes:  In hardware these blocks become top level output ports or are discarded, depending on how they are configured."  xl_area=[0 0 0 0 0 0 0]  block_version=10.1.3
  Logical : xbsIndex_r4/Logical  logical_function=XOR  inputs=3  en=off  latency=1  precision=Full  arith_type=Unsigned  n_bits=8  bin_pt=2  align_bp=off  dbl_ovrd=off  block_type=logical
      settings: xl_area=[32 32 0 32 0 0 0]
  Mux : xbsIndex_r4/Mux  inputs=2  en=off  latency=1  precision=Full  arith_type="Signed  (2's comp)"  n_bits=8  bin_pt=2  quantization=Truncate  overflow=Wrap  dbl_ovrd=off  block_type=mux
      settings: xl_area=[16 32 0 32 0 0 0]
  Mux1 : xbsIndex_r4/Mux  inputs=2  en=off  latency=1  precision=Full  arith_type="Signed  (2's comp)"  n_bits=8  bin_pt=2  quantization=Truncate  overflow=Wrap  dbl_ovrd=off  block_type=mux
      settings: xl_area=[16 32 0 32 0 0 0]
  Scope : Scope  NumInputPorts=4
      settings: YMin=-5~-5~-5~-5  YMax=5~5~5~5
  a : xbsIndex_r4/Constant  const=hex2dec('8EBFD028')  gui_display_data_type=Fixed-point  arith_type=Unsigned  n_bits=32  bin_pt=0  preci_type=Single  exp_width=8  frac_width=24  explicit_period=off  period=1  equ=P=C  opselect=C  inp2=PCIN>>17  opr=+  inp1=P  carry=CIN  dbl_ovrd=off  block_type=constant
  delay : xbsIndex_r4/Delay  rst=off  infoeditControl=Selection of Reset will increase slice count due to use of real FFs and instead of SRLs  en=off  latency=1  dbl_ovrd=off  reg_retiming=off  block_type=delay
      settings: xl_area=[16 32 0 0 0 0 0]
  lsb : xbsIndex_r4/Slice  nbits=1  boolean_output=off  mode=Lower Bit Location + Width  bit1=0  base1=MSB of Input  bit0=0  base0=LSB of Input  dbl_ovrd=off  block_type=slice
      settings: infoedit="Extracts a given range of bits from each input sample and presents it at the output.  The output type is ordinarily unsigned with binary point at zero, but can be Boolean when the slice is one bit wide.<P><P>Hardware notes: In hardware this block costs nothing."  block_version=10.1.3
  output : Subsystem
  rshift_1 : xbsIndex_r4/Shift  shift_dir=Right  shift_bits=1  en=off  latency=1  precision=User Defined  arith_type=Unsigned  n_bits=32  bin_pt=0  quantization=Truncate  overflow=Wrap  dbl_ovrd=off  block_type=shift
      settings: xl_area=[0 32 0 0 0 0 0]  block_version=10.1.3
  x_l : xbsIndex_r4/Delay  rst=off  infoeditControl=Selection of Reset will increase slice count due to use of real FFs and instead of SRLs  en=off  latency=7  dbl_ovrd=off  reg_retiming=off  block_type=delay
      settings: xl_area=[16 32 0 32 0 0 0]
  x_l_m : xbsIndex_r4/Delay  rst=off  infoeditControl=Selection of Reset will increase slice count due to use of real FFs and instead of SRLs  en=off  latency=25-7-3  dbl_ovrd=off  reg_retiming=off  block_type=delay
      settings: xl_area=[16 32 0 32 0 0 0]
  u : Outport
  wires:
  delay/1 -> Logical/1
  output/1(out) -> u/1
  Gateway Out3/1 -> Scope/4
  Gateway Out2/1 -> Scope/3
  Gateway Out4/1 -> Scope/2
  Gateway Out1/1 -> Scope/1
  seed/1 -> Mux1/3, Gateway Out4/1
  seed_en/1 -> Mux1/1, Gateway Out1/1
  Mux1/1 -> Gateway Out2/1, x_l_m/1
  Logical/1 -> Mux1/2, Gateway Out3/1
  Mux/1 -> Logical/3
  rshift_1/1 -> Logical/2
  a/1 -> Mux/3
  Constant3/1 -> Mux/2
  lsb/1 -> Mux/1
  x_l/1 -> output/1(in), rshift_1/1, lsb/1
  x_l_m/1 -> delay/1, x_l/1

== system r2_deng_rev1_13_wide/wng_corr/wgn3/tt800_uprng/tt800_seed_gen ==
  seed_in : Inport
  ld : Inport  Port=2
  rst : Inport  Port=3
  Expression : xbsIndex_r4/Expression  expression=(bootstrap | ld | ld_ext)  align_bp=on  en=off  latency=1  precision=Full  arith_type=Unsigned  n_bits=8  bin_pt=2  dbl_ovrd=off  block_type=expr
      settings: xl_area=[0, 0, 0, 0, 0, 0, 0]  block_version=10.1.3
  LFSR : xbsIndex_r4/LFSR  lfsr_type=Fibonacci  gate_type=XOR  n_bits=32  polynomial='C0000401'  rst_value='98321495'  rst=on  en=off  reloadable_seed=on  input_type=on  output_type=on  arith_type=Unsigned  bin_pt=0  dbl_ovrd=off  explicit_period=on  period=1  block_type=lfsr
      settings: xl_area=[17 32 0 33 0 0 0]  block_version=10.1.3
  bootstrap : Subsystem
  p24_extender : Subsystem
  pipeline1 : Subsystem  AncestorBlock=casper_library_delays/pipeline  mask(pipeline){latency=2}
      mask help:
      | An explicitly laid-out delay line to avoid mapping to SRL16s
      | for use in pipelining to help achieve timing closure.
      mask init:
      | pipeline_init(gcb,'latency',latency);
      settings: AttributesFormatString=Latency = %<latency>
      mask Display:
      | port_label('input', 1, 'd');
      | port_label('output', 1, 'q');
      | disp(['Z^-', num2str(latency)]);
  pipeline2 : Subsystem  AncestorBlock=casper_library_delays/pipeline  mask(pipeline){latency=2}
      mask help:
      | An explicitly laid-out delay line to avoid mapping to SRL16s
      | for use in pipelining to help achieve timing closure.
      mask init:
      | pipeline_init(gcb,'latency',latency);
      settings: AttributesFormatString=Latency = %<latency>
      mask Display:
      | port_label('input', 1, 'd');
      | port_label('output', 1, 'q');
      | disp(['Z^-', num2str(latency)]);
  r_edge_detect : Subsystem
  seed_out : Outport
  seed_en : Outport  Port=2
  wires:
  r_edge_detect/1(out) -> p24_extender/1(in)
  ld/1 -> LFSR/2, r_edge_detect/1(in), Expression/2
  Expression/1 -> seed_en/1
  seed_in/1 -> LFSR/1
  LFSR/1 -> seed_out/1
  bootstrap/1(out) -> Expression/1
  p24_extender/1(out) -> Expression/3
  rst/1 -> pipeline1/1(d), pipeline2/1(d), LFSR/3
  pipeline1/1(q) -> p24_extender/2(rst)
  pipeline2/1(q) -> bootstrap/1(rst)
